simulink model "tallerInt1SMLK"  (R2020b)
settings: Solver=VariableStepAuto  StartTime=0.0  StopTime=10.0  RelTol=1e-3
undefined symbols (not defined in the file): mod
libraries: simulink x2
settings Model: Creator=andre  LastModifiedBy=andre

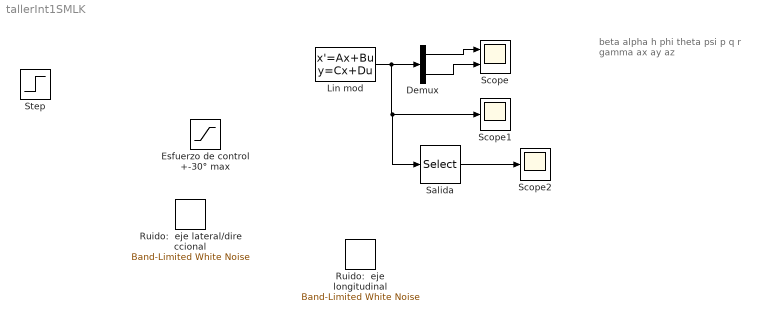
== system tallerInt1SMLK ==
  note: beta
      | alpha
      | h
      | phi
      | theta
      | psi
      | p
      | q
      | r
      | gamma
      | ax
      | ay
      | az
  Demux : Demux  Outputs=2
  Esfuerzo de control +-30° max : Saturate  UpperLimit=30  LowerLimit=-30
  Lin mod : StateSpace  A=mod.A  B=mod.B  C=mod.C  D=mod.D  InitialCondition=0
  Ruido:  eje lateral/direccional : simulink/Sources/Band-Limited White Noise  Cov=[0.001]  Ts=0.1  seed=[23341]
  Ruido:  eje longitudinal : simulink/Sources/Band-Limited White Noise  Cov=[0.001]  Ts=0.1  seed=[23341]
  Salida : Selector  InputPortWidth=14  IndexOptions=Index vector (dialog)  Indices=[5 6]  OutputSizes=1
  Scope : Scope  NumInputPorts=2
  Scope1 : Scope
  Scope2 : Scope
  Step : Step  SampleTime=0
  wires:
  Lin mod/1 -> Salida/1, Scope1/1, Demux/1
  Demux/1 -> Scope/1
  Demux/2 -> Scope/2
  Salida/1 -> Scope2/1
